simulink model "llc_converter"  (R2022b)
settings: Solver=ode23t  StartTime=0.0  StopTime=1e-3  RelTol=1e-3
values from neighbouring files (symbols this model uses):
  td = 1.5e-07    [param.mat]
  Ts = 1.17647058824e-05    [param.mat]
libraries: spsSeriesRLCBranchLib x5, spsVoltageMeasurementLib x4, spsCurrentMeasurementLib x2, spsDiodeLib x2, spsGroundLib x2, spsMosfetLib x2, spsDCVoltageSourceLib x1, spsFourierLib x1, spsLinearTransformerLib x1, spsMeanLib x1, spsRMSLib x1, sps_lib x1
settings Model: Creator=Ilya  LastModifiedBy=Ilya

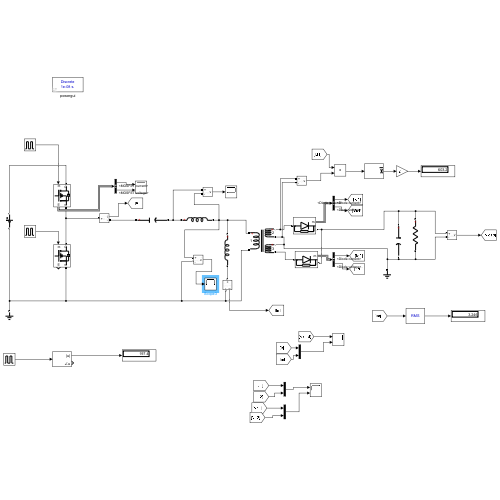
[thumbnail: Simulink's stored preview of the top-level diagram]
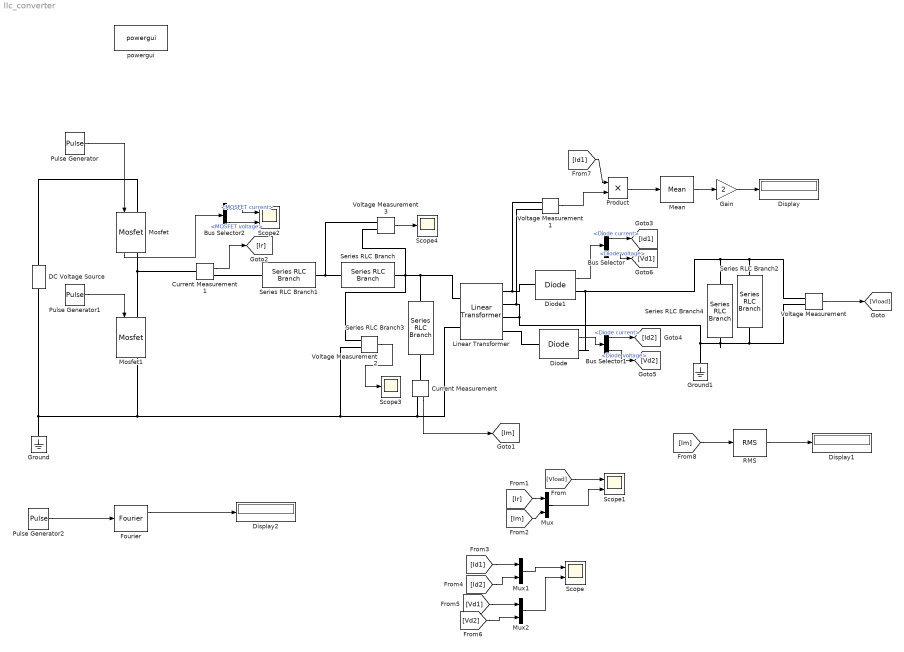
== system llc_converter ==
  Bus Selector : BusSelector  OutputSignals=Diode current,Diode voltage
  Bus Selector1 : BusSelector  OutputSignals=Diode current,Diode voltage
  Bus Selector2 : BusSelector  OutputSignals=MOSFET current,MOSFET voltage
  Current Measurement : spsCurrentMeasurementLib/Current Measurement  PhasorSimulation=off  OutputType=Complex  PSBequivalent=0
  Current Measurement1 : spsCurrentMeasurementLib/Current Measurement  PhasorSimulation=off  OutputType=Complex  PSBequivalent=0
  DC Voltage Source : spsDCVoltageSourceLib/DC Voltage Source  Amplitude=310  Measurements=None
  Diode : spsDiodeLib/Diode  Ron=0.001  Lon=0  Vf=0.5  IC=0  UseSnubber=0  Rs=500  Cs=250e-9  Measurements=on
  Diode1 : spsDiodeLib/Diode  Ron=0.001  Lon=0  Vf=0.5  IC=0  UseSnubber=0  Rs=500  Cs=250e-9  Measurements=on
  Display : Display
  Display1 : Display
  Display2 : Display
  Fourier : spsFourierLib/Fourier  Freq=Fs  n=1  InInit=[0, 0]  Ts=0
  Gain : Gain  Gain=2
  Ground : spsGroundLib/Ground  LConnTagsString=a
  Ground1 : spsGroundLib/Ground  LConnTagsString=a
  Linear Transformer : spsLinearTransformerLib/Linear Transformer  UNITS=SI  NominalPower=[1500 150e3 ]  winding1=[7 0 0]  winding2=[1 0 0]  ThreeWindings=on  winding3=[1 0 0]  RmLm=[1.0804e+06 0]  Measurements=None  DataType=on
  Mean : spsMeanLib/Mean  Freq=115e3  Vinit=0  Ts=0
  Mosfet : spsMosfetLib/Mosfet  Ron=0.29  Lon=0  Rd=0.01  Vfd=1.5  IC=0  Rs=1e5  Cs=inf  Measurements=on
  Mosfet1 : spsMosfetLib/Mosfet  Ron=0.29  Lon=0  Rd=0.01  Vfd=1.5  IC=0  Rs=1e5  Cs=inf  Measurements=on
  Mux : Mux  Inputs=2
  Mux1 : Mux  Inputs=2
  Mux2 : Mux  Inputs=2
  Product : Product
  Pulse Generator : DiscretePulseGenerator  PulseType=Time based  Period=Ts  PulseWidth=(Ts/2-td)/Ts*100
  Pulse Generator1 : DiscretePulseGenerator  PulseType=Time based  Period=Ts  PulseWidth=(Ts/2-td)/Ts*100  PhaseDelay=Ts/2
  Pulse Generator2 : DiscretePulseGenerator  PulseType=Time based  Amplitude=310  Period=Ts  PulseWidth=50
  RMS : spsRMSLib/RMS  TrueRMS=on  Freq=115e3  RMSInit=0  Ts=0
  Scope : Scope  NumInputPorts=2
  Scope1 : Scope  NumInputPorts=2
  Scope2 : Scope  NumInputPorts=2
  Scope3 : Scope
  Scope4 : Scope
  Series RLC Branch : spsSeriesRLCBranchLib/Series RLC Branch  LConnTagsString=__new0  RConnTagsString=__new0  BranchType=L  Resistance=1  Inductance=22e-6  SetiL0=off  InitialCurrent=0  Capacitance=1e-6  Setx0=off  InitialVoltage=0  Measurements=None
  Series RLC Branch1 : spsSeriesRLCBranchLib/Series RLC Branch  LConnTagsString=__new0  RConnTagsString=__new0  BranchType=C  Resistance=1  Inductance=22e-6  SetiL0=off  InitialCurrent=0  Capacitance=67e-9  Setx0=off  InitialVoltage=0  Measurements=None
  Series RLC Branch2 : spsSeriesRLCBranchLib/Series RLC Branch  LConnTagsString=__new0  RConnTagsString=__new0  BranchType=R  Resistance=1  Inductance=22e-6  SetiL0=off  InitialCurrent=0  Capacitance=1e-6  Setx0=off  InitialVoltage=0  Measurements=None
  Series RLC Branch3 : spsSeriesRLCBranchLib/Series RLC Branch  LConnTagsString=__new0  RConnTagsString=__new0  BranchType=L  Resistance=1  Inductance=66e-6  SetiL0=off  InitialCurrent=0  Capacitance=1e-6  Setx0=off  InitialVoltage=0  Measurements=None
  Series RLC Branch4 : spsSeriesRLCBranchLib/Series RLC Branch  LConnTagsString=__new0  RConnTagsString=__new0  BranchType=C  Resistance=1  Inductance=66e-6  SetiL0=off  InitialCurrent=0  Capacitance=200e-6  Setx0=off  InitialVoltage=0  Measurements=None
  Voltage Measurement{,1..3} (4 alike) : spsVoltageMeasurementLib/Voltage Measurement  PhasorSimulation=off  OutputType=Complex  PSBequivalent=0
  powergui : sps_lib/powergui  Priority=1  SimulationMode=Discrete  SampleTime=1e-8  frequency=60  Iterations=50  frequencyindice=0  Pbase=100e6  ErrMax=1e-4  UnitsV=kV  UnitsW=MW  buscounter=0  FunctionMessages=off  echomessages=off  EnableUseOfTLC=off  CurrentSourceSwitches=off  DisableSnubberDevices=off  DisableRonSwitches=off  DisableVfSwitches=off  DisplayEquations=off  AutomaticDiscreteSolvers=off  SolverType=Tustin/Backward Euler (TBE)  Interpol=off  ExternalGateDelay=off  methode=off  Ts=100  x0status=blocks  SPID=on  SwTol=0  HookPort=off  NonlinearTolerance=1e-4  nMaxIteration=100  ContinueOnMaxIteration=off  RestoreLinks=warning  ResistiveCurrentMeasurement=off  Frange=[0:2:500]  Ylog=off  Xlog=on  ShowGrid=off  save=off  variable=ZData  structure=0  ZoomFFT=off  StartTime=0.0  cycles=1  DisplayStyle=1  fundamental=60  FreqAxis=off  MaxFrequency=1000  frequencyindicesteady=1  RmsSteady=1  display=off
  wires:
  Pulse Generator/1 -> Mosfet/1
  Pulse Generator1/1 -> Mosfet1/1
  Voltage Measurement/1 -> [Vload]
  Current Measurement/1 -> [Im]
  Current Measurement1/1 -> [Ir]
  [Vload] -> Scope1/1
  [Ir] -> Mux/1
  [Im] -> Mux/2
  Mux/1 -> Scope1/2
  Diode1/1 -> Bus Selector/1
  Diode/1 -> Bus Selector1/1
  Bus Selector/1 -> [Id1]  "<Diode current>"
  Bus Selector1/1 -> [Id2]  "<Diode current>"
  Bus Selector1/2 -> [Vd2]  "<Diode voltage>"
  Bus Selector/2 -> [Vd1]  "<Diode voltage>"
  [Id1] -> Mux1/1
  [Id2] -> Mux1/2
  Mux1/1 -> Scope/1
  [Vd1] -> Mux2/1
  [Vd2] -> Mux2/2
  Mux2/1 -> Scope/2
  Mosfet/1 -> Bus Selector2/1
  Bus Selector2/1 -> Scope2/1  "<MOSFET current>"
  Bus Selector2/2 -> Scope2/2  "<MOSFET voltage>"
  [Id1] -> Product/1
  Voltage Measurement1/1 -> Product/2
  Mean/1 -> Gain/1
  Product/1 -> Mean/1
  Gain/1 -> Display/1
  Voltage Measurement2/1 -> Scope3/1
  Voltage Measurement3/1 -> Scope4/1
  [Im] -> RMS/1
  RMS/1 -> Display1/1
  Pulse Generator2/1 -> Fourier/1
  Fourier/1 -> Display2/1
  connections:
  Ground/LConn1 -- Mosfet1/RConn1 -- Voltage Measurement2/LConn2 -- Current Measurement/RConn1 -- Linear Transformer/LConn2 -- DC Voltage Source/LConn1
  Mosfet1/LConn1 -- Current Measurement1/LConn1 -- Mosfet/RConn1
  Series RLC Branch/LConn1 -- Voltage Measurement3/LConn1 -- Series RLC Branch1/RConn1
  Series RLC Branch/RConn1 -- Voltage Measurement3/LConn2 -- Voltage Measurement2/LConn1 -- Series RLC Branch3/LConn1 -- Linear Transformer/LConn1
  Series RLC Branch2/RConn1 -- Voltage Measurement/LConn2 -- Series RLC Branch4/RConn1 -- Linear Transformer/RConn3 -- Voltage Measurement1/LConn2 -- Linear Transformer/RConn2 -- Ground1/LConn1
  Diode/LConn1 -- Linear Transformer/RConn4
  Linear Transformer/RConn1 -- Voltage Measurement1/LConn1 -- Diode1/LConn1
  Diode/RConn1 -- Series RLC Branch4/LConn1 -- Voltage Measurement/LConn1 -- Series RLC Branch2/LConn1 -- Diode1/RConn1
  Mosfet/LConn1 -- DC Voltage Source/RConn1
  Current Measurement/LConn1 -- Series RLC Branch3/RConn1
  Series RLC Branch1/LConn1 -- Current Measurement1/RConn1
